simulink model "test"  (R2018b)
settings: Solver=VariableStepAuto  StartTime=0.0  StopTime=20  FixedStep=Ts  RelTol=1e-9
values from neighbouring files (symbols this model uses):
  loadVelocity = reshape(loadVelocity, [1, 3])    [EvaluateTrajectory.m]    (also in evaluationTest.m = [1e-3 1e-3 1e-3])
  numOfPoints = length(refPointsVector)/3    [EvaluateTrajectory.m]    (also in evaluationTest.m)
  refPointsVector = [0 0 0 0.5 0 0 1 0 0]    [evaluationTest.m]
  Ts = 0.05    [evaluationTest.m]
undefined symbols (not defined in the file or in its folder): EvaluateTrajectory
settings Model: Creator=Marko  LastModifiedBy=Marko

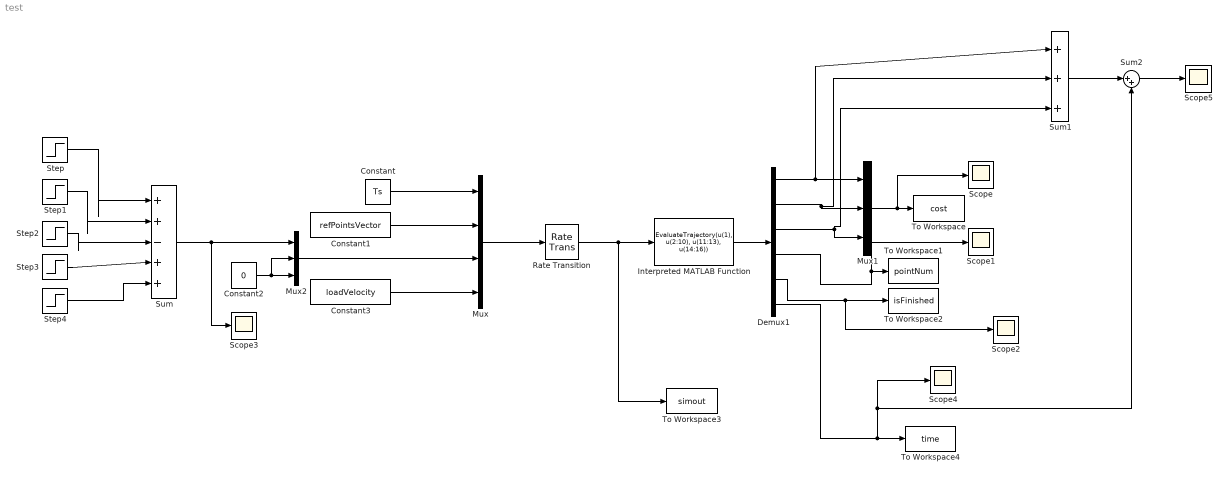
== system test ==
  Constant : Constant  Value=Ts  SampleTime=Ts
  Constant1 : Constant  Value=refPointsVector  SampleTime=Ts
  Constant2 : Constant  Value=0
  Constant3 : Constant  Value=loadVelocity  SampleTime=Ts
  Demux1 : Demux  Outputs=6
  Interpreted MATLAB Function : MATLABFcn  MATLABFcn=EvaluateTrajectory(u(1), u(2:10), u(11:13), u(14:16))  OutputDimensions=numOfPoints+3  OutputSignalType=real
  Mux : Mux
  Mux1 : Mux  Inputs=3
  Mux2 : Mux  Inputs=3
  Rate Transition : RateTransition  OutPortSampleTime=Ts
  Scope{,1..5} (6 alike) : Scope
  Step : Step  Time=2  Before=-0.5  After=0.05  SampleTime=0
  Step1 : Step  Time=5  After=0.5  SampleTime=0
  Step2 : Step  Time=5.5  After=0.5  SampleTime=0
  Step3 : Step  Time=8  After=0.5  SampleTime=0
  Step4 : Step  Time=15  After=0.5  SampleTime=0
  Sum : Sum  Inputs=|++-++
  Sum1 : Sum  Inputs=|+++
  Sum2 : Sum  Inputs=|++
  To Workspace : ToWorkspace  VariableName=cost  SampleTime=Ts
  To Workspace1 : ToWorkspace  VariableName=pointNum  SampleTime=Ts
  To Workspace2 : ToWorkspace  VariableName=isFinished  SampleTime=Ts
  To Workspace3 : ToWorkspace  VariableName=simout  SampleTime=Ts
  To Workspace4 : ToWorkspace  VariableName=time  SampleTime=Ts
  wires:
  Constant1/1 -> Mux/2
  Demux1/1 -> Sum1/1, Mux1/1
  Demux1/2 -> Mux1/2, Sum1/2
  Demux1/3 -> Sum1/3, Mux1/3
  Constant/1 -> Mux/1
  Mux2/1 -> Mux/3
  Constant3/1 -> Mux/4
  Constant2/1 -> Mux2/2, Mux2/3
  Step/1 -> Sum/1
  Sum/1 -> Scope3/1, Mux2/1
  Step1/1 -> Sum/2
  Demux1/4 -> Scope1/1, To Workspace1/1
  Demux1/5 -> Scope2/1, To Workspace2/1
  Step2/1 -> Sum/3
  Step3/1 -> Sum/4
  Step4/1 -> Sum/5
  Interpreted MATLAB Function/1 -> Demux1/1
  Mux1/1 -> Scope/1, To Workspace/1
  Sum1/1 -> Sum2/1
  Demux1/6 -> Sum2/2, Scope4/1, To Workspace4/1
  Sum2/1 -> Scope5/1
  Mux/1 -> Rate Transition/1
  Rate Transition/1 -> To Workspace3/1, Interpreted MATLAB Function/1
